simulink model "schemat"  (R2025b)
settings: Solver=VariableStepAuto  StartTime=0.0  StopTime=100.0  RelTol=1e-3
values from neighbouring files (symbols this model uses):
  A = 7    [PID.m]    (also in zadanie.m)
  B = 5    [PID.m]    (also in zadanie.m)
libraries: simulink x1, slpidlib x1
settings Model: Creator=andos  LastModifiedBy=andos

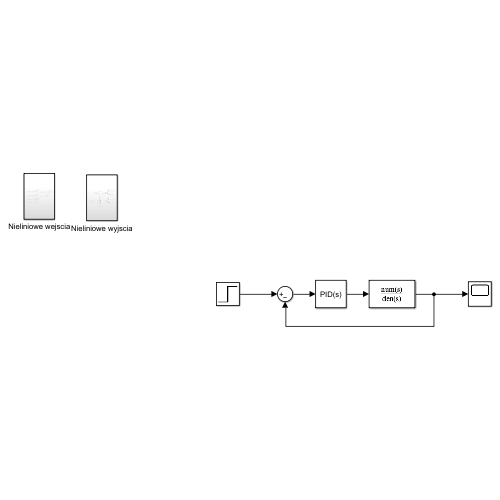
[thumbnail: Simulink's stored preview of the top-level diagram]
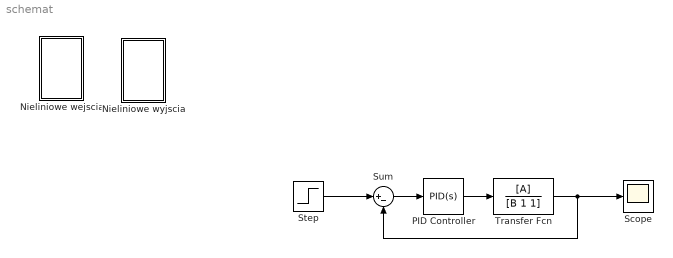
== system schemat ==
  Nieliniowe wejscia : Subsystem
  Nieliniowe wyjscia : Subsystem
  PID Controller : slpidlib/PID Controller  Controller=PID  Form=Parallel  TimeDomain=Continuous-time  UseExternalTs=off  SampleTime=-1  IntegratorMethod=Forward Euler  FilterMethod=Forward Euler  ControllerParametersSource=internal  P=4  I=2  UseKiTs=off  D=3.76  UseExternalDerivativeSource=off  N=100  UseFilter=on  TunerSelectOption=Transfer Function Based (PID Tuner App)  InitialConditionSource=internal  InitialConditionForIntegrator=0  InitialConditionForFilter=0  DifferentiatorICPrevScaledInput=0  ExternalReset=none  TrackingMode=off  Kt=1  LimitOutput=off  SatLimitsSource=internal  UpperSaturationLimit=inf  LowerSaturationLimit=-inf  LinearizeAsGain=on  AntiWindupMode=none  Kb=1  LimitIntegrator=off  UpperIntegratorSaturationLimit=inf  LowerIntegratorSaturationLimit=-inf  POutMin=[]  POutMax=[]  IOutMin=[]  IOutMax=[]  DOutMin=[]  DOutMax=[]  NOutMin=[]  NOutMax=[]  SumOutMin=[]  SumOutMax=[]  SaturationOutMin=[]  SaturationOutMax=[]  PParamMin=[]  PParamMax=[]  IParamMin=[]  IParamMax=[]  DParamMin=[]  DParamMax=[]  NParamMin=[]  NParamMax=[]  KbParamMin=[]  KbParamMax=[]  KtParamMin=[]  KtParamMax=[]  KbOutMin=[]  KbOutMax=[]  KtOutMin=[]  KtOutMax=[]  IntegratorOutMin=[]  IntegratorOutMax=[]  FilterOutMin=[]  FilterOutMax=[]  SumI1OutMin=[]  SumI1OutMax=[]  SumI2OutMin=[]  SumI2OutMax=[]  SumI3OutMin=[]  SumI3OutMax=[]  SumI4OutMin=[]  SumI4OutMax=[]  SumDOutMin=[]  SumDOutMax=[]  DifferentiatorOutMin=[]  DifferentiatorOutMax=[]  FilterDiffOutCoefMin=[]  FilterDiffOutCoefMax=[]  ReciprocalOutMin=[]  ReciprocalOutMax=[]  SumDenOutMin=[]  SumDenOutMax=[]  SumNumOutMin=[]  SumNumOutMax=[]  DivideOutMin=[]  DivideOutMax=[]  UdiffTsProdOutMin=[]  UdiffTsProdOutMax=[]  NTsProdOutMin=[]  NTsProdOutMax=[]  UintegralTsProdOutMin=[]  UintegralTsProdOutMax=[]  UngainTsProdOutMin=[]  UngainTsProdOutMax=[]  ClampingZeroOutDataTypeStr=Inherit: Inherit via back propagation  ClampingZeroOutMin=[]  ClampingZeroOutMax=[]  FilterDenConstantOutDataTypeStr=Inherit: Inherit via back propagation  FilterDenConstantOutMin=[]  FilterDenConstantOutMax=[]  PCopyOutDataTypeStr=Inherit: Inherit via back propagation  PCopyOutMin=[]  PCopyOutMax=[]  NCopyOutDataTypeStr=Inherit: Inherit via back propagation  NCopyOutMin=[]  NCopyOutMax=[]  IntegratorContinuousStateAttributes=''  IntegratorStateMustResolveToSignalObject=off  IntegratorRTWStateStorageClass=Auto  FilterContinuousStateAttributes=''  FilterStateMustResolveToSignalObject=off  FilterRTWStateStorageClass=Auto  ParallelPVariant=InternalParameters  IdealPVariant=Disabled  IVariant=InternalParameters  DVariant=InternalParameters  IntegratorVariant=Continuous  SatVariant=Disabled  AWVariant=Passthrough  PCopyVariant=Disabled  TRVariant=Disabled  FdbkBlocksVariant=Forward  IdealPFdbkVariant=Disabled  SatFdbkVariant=Disabled  DerivativeFilterVariant=ContFilter  NVariant=InternalParameters  NCopyVariant=Disabled  FilterICVariant=InternalICsFilter  IntegratorICVariant=InternalICs  ExternalResetVariant=Disabled  TRSumVariant=Passthrough  SumFdbkVariant=Disabled  SumVariant=Sum_PID  TsampFilterVariant=InternalTs  TsampNgainVariant=Passthrough  TsampIntegralVariant=Disabled_SignalSpec  ExternalSaturationOutDataTypeStr=Inherit: Same as second input  DerivativeSourceVariant=ErrorSignal  PreIntVariant=InternalPreInt
  Scope : Scope
      settings: ActiveDisplayYMinimum=-6.8363257388752222E+8  ActiveDisplayYMaximum=2.2948740257197089E+9  DataLoggingVariableName=ScopeData8
  Step : Step  After=5  SampleTime=0
  Sum : Sum  Inputs=|+-
  Transfer Fcn : TransferFcn  Numerator=[A]  Denominator=[B 1 1]
  wires:
  Step/1 -> Sum/1
  Sum/1 -> PID Controller/1
  PID Controller/1 -> Transfer Fcn/1
  Transfer Fcn/1 -> Scope/1, Sum/2

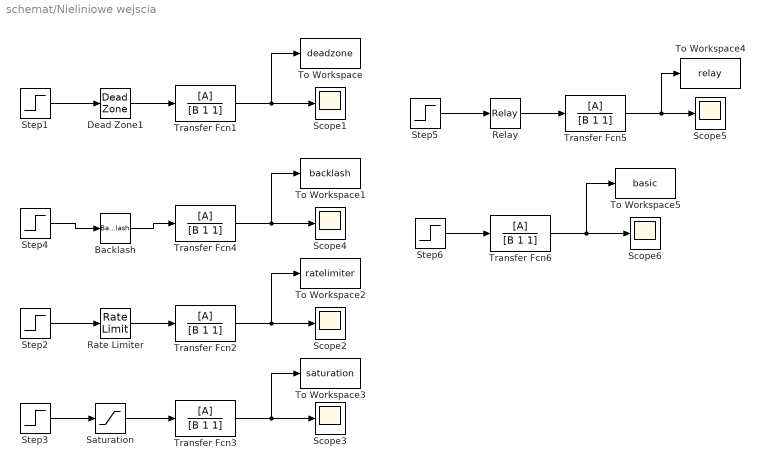
== system schemat/Nieliniowe wejscia ==
  Backlash : Backlash
  Dead Zone1 : DeadZone
  Rate Limiter : RateLimiter  SampleTimeMode=inherited
  Relay : Relay
  Saturation : Saturate
  Scope{1..6} (6 alike) : Scope
      Scope1 settings: ActiveDisplayYMinimum=-1.2979978301894766  ActiveDisplayYMaximum=11.681980471705291
      Scope2 settings: ActiveDisplayYMinimum=-1.2979978301894766  ActiveDisplayYMaximum=11.681980471705291  DataLoggingVariableName=ScopeData2
      Scope3 settings: ActiveDisplayYMinimum=-1.2979978301894766  ActiveDisplayYMaximum=11.681980471705291  DataLoggingVariableName=ScopeData3
      Scope4 settings: ActiveDisplayYMinimum=-1.2979978301894766  ActiveDisplayYMaximum=11.681980471705291
      Scope5 settings: ActiveDisplayYMinimum=-1.2979978301894766  ActiveDisplayYMaximum=11.681980471705291  DataLoggingVariableName=ScopeData4
      Scope6 settings: ActiveDisplayYMinimum=-1.2979978301894766  ActiveDisplayYMaximum=11.681980471705291  DataLoggingVariableName=ScopeData5
  Step{1..6} (6 alike) : Step  SampleTime=0
  To Workspace : ToWorkspace  VariableName=deadzone  SampleTime=-1
  To Workspace1 : ToWorkspace  VariableName=backlash  SampleTime=-1
  To Workspace2 : ToWorkspace  VariableName=ratelimiter  SampleTime=-1
  To Workspace3 : ToWorkspace  VariableName=saturation  SampleTime=-1
  To Workspace4 : ToWorkspace  VariableName=relay  SampleTime=-1
  To Workspace5 : ToWorkspace  VariableName=basic  SampleTime=-1
  Transfer Fcn{1..6} (6 alike) : TransferFcn  Numerator=[A]  Denominator=[B 1 1]
  wires:
  Dead Zone1/1 -> Transfer Fcn1/1
  Transfer Fcn4/1 -> To Workspace1/1, Scope4/1
  Step1/1 -> Dead Zone1/1
  Transfer Fcn1/1 -> To Workspace/1, Scope1/1
  Transfer Fcn6/1 -> To Workspace5/1, Scope6/1
  Backlash/1 -> Transfer Fcn4/1
  Step4/1 -> Backlash/1
  Step3/1 -> Saturation/1
  Step2/1 -> Rate Limiter/1
  Rate Limiter/1 -> Transfer Fcn2/1
  Step6/1 -> Transfer Fcn6/1
  Transfer Fcn5/1 -> To Workspace4/1, Scope5/1
  Transfer Fcn2/1 -> To Workspace2/1, Scope2/1
  Saturation/1 -> Transfer Fcn3/1
  Transfer Fcn3/1 -> To Workspace3/1, Scope3/1
  Relay/1 -> Transfer Fcn5/1
  Step5/1 -> Relay/1

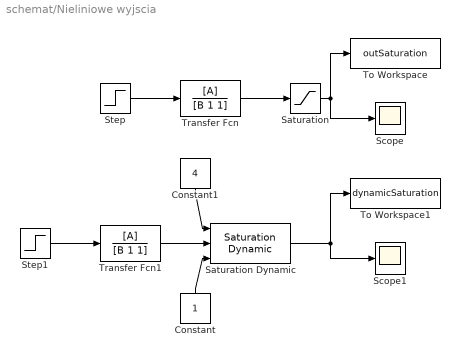
== system schemat/Nieliniowe wyjscia ==
  Constant : Constant
  Constant1 : Constant  Value=4
  Saturation : Saturate
  Saturation Dynamic : simulink/Discontinuities/Saturation Dynamic  OutMin=[]  OutMax=[]  OutDataTypeStr=Inherit: Same as second input  OutDataType=fixdt(1, 16)  OutScaling=2^-10  DoSatur=off
  Scope : Scope
      settings: ActiveDisplayYMinimum=-0.062499999999999986  ActiveDisplayYMaximum=0.5625  DataLoggingVariableName=ScopeData6
  Scope1 : Scope
      settings: ActiveDisplayYMinimum=1.3480885311871229  ActiveDisplayYMaximum=5  DataLoggingVariableName=ScopeData7
  Step : Step  SampleTime=0
  Step1 : Step  SampleTime=0
  To Workspace : ToWorkspace  VariableName=outSaturation  SampleTime=-1
  To Workspace1 : ToWorkspace  VariableName=dynamicSaturation  SampleTime=-1
  Transfer Fcn : TransferFcn  Numerator=[A]  Denominator=[B 1 1]
  Transfer Fcn1 : TransferFcn  Numerator=[A]  Denominator=[B 1 1]
  wires:
  Saturation/1 -> Scope/1, To Workspace/1
  Saturation Dynamic/1 -> To Workspace1/1, Scope1/1
  Step/1 -> Transfer Fcn/1
  Step1/1 -> Transfer Fcn1/1
  Transfer Fcn1/1 -> Saturation Dynamic/2
  Constant1/1 -> Saturation Dynamic/1
  Constant/1 -> Saturation Dynamic/3
  Transfer Fcn/1 -> Saturation/1
